simulink model "model5"  (R2022b)
settings: Solver=ode3  StartTime=0.0  StopTime=10  FixedStep=0.0005  RelTol=1e-3
values from neighbouring files (symbols this model uses):
  a21 = 1/2/m * x30^2 * FemP1/FemP2^2 * exp(-x10/FemP2)    [init.m]    (also in proj.m)
  a23 = -1/m * x30 * FemP1/FemP2 * exp(-x10/FemP2)    [init.m]    (also in proj.m)
  a31 = 1/f1 * exp(x10/f2) * (ki*u10 + ci - x30)    [init.m]    (also in proj.m)
  a33 = -f2/f1 * exp(x10/f2)    [init.m]    (also in proj.m)
  b31 = ki * f2/f1 * exp(x10/f2)    [init.m]    (also in proj.m)
  g = 9.81    [init.m]    (also in proj.m)
  K = place(A, B(:, 1), [-28, -60, -90])    [init.m]    (also in proj.m)
  L = acker(A', C', p)'    [init.m]    (also in proj.m)
  u10 = 1/ki*(x30-ci)    [init.m]    (also in proj.m)
  xd = d-bd    [init.m]    (also in proj.m)
settings Model: Creator=TheZl  LastModifiedBy=TheZl

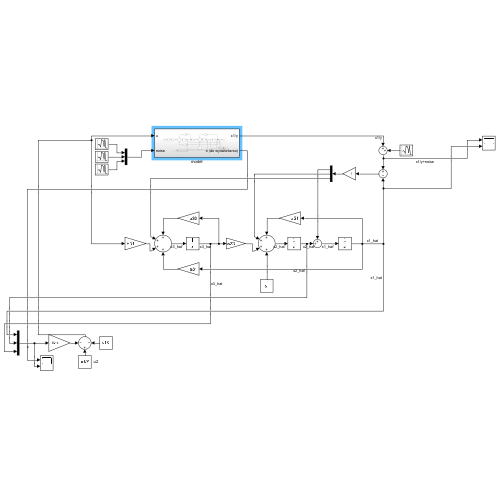
[thumbnail: Simulink's stored preview of the top-level diagram]
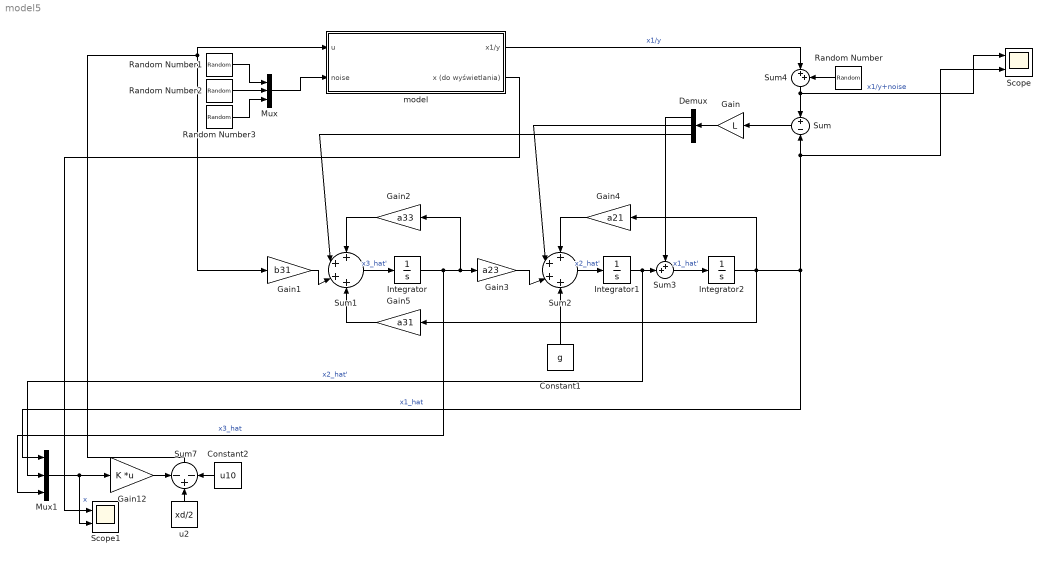
== system model5 ==
  Constant1 : Constant  Value=g
  Constant2 : Constant  Value=u10
  Demux : Demux  Outputs=3
  Gain : Gain  Gain=L
  Gain1 : Gain  Gain=b31
  Gain12 : Gain  Gain=K  Multiplication=Matrix(K*u)
  Gain2 : Gain  Gain=a33
  Gain3 : Gain  Gain=a23
  Gain4 : Gain  Gain=a21
  Gain5 : Gain  Gain=a31
  Integrator : Integrator
  Integrator1 : Integrator
  Integrator2 : Integrator  UpperSaturationLimit=xd  LowerSaturationLimit=0
  Mux : Mux  Inputs=3
  Mux1 : Mux  Inputs=3
  Random Number : RandomNumber  Variance=1e-5
  Random Number1 : RandomNumber  Variance=1e-5
  Random Number2 : RandomNumber  Variance=1e-5
  Random Number3 : RandomNumber  Variance=1e-2
  Scope : Scope  NumInputPorts=2
  Scope1 : Scope  NumInputPorts=2
  Sum : Sum  Inputs=+|-
  Sum1 : Sum  Inputs=++++
  Sum2 : Sum  Inputs=++++
  Sum3 : Sum  Inputs=++|
  Sum4 : Sum  Inputs=|++
  Sum7 : Sum  Inputs=-+-
  model : Subsystem
  u2 : Constant  Value=xd/2
  wires:
  model/1(x1/y) -> Sum4/1  "x1/y"
  Sum/1 -> Gain/1
  Sum7/1 -> Gain1/1, model/1(u)
  Gain4/1 -> Sum2/1
  Sum2/1 -> Integrator1/1  "x2_hat'"
  Sum1/1 -> Integrator/1  "x3_hat'"
  Constant1/1 -> Sum2/4
  Gain5/1 -> Sum1/4
  Gain2/1 -> Sum1/1
  Gain/1 -> Demux/1
  Demux/2 -> Sum2/2
  Gain3/1 -> Sum2/3
  Gain1/1 -> Sum1/3
  Sum3/1 -> Integrator2/1  "x1_hat'"
  Demux/1 -> Sum3/1
  Demux/3 -> Sum1/2
  Integrator2/1 -> Gain4/1, Mux1/1, Sum/2, Scope/2, Gain5/1  "x1_hat"
  Integrator/1 -> Mux1/3, Gain2/1, Gain3/1  "x3_hat"
  Integrator1/1 -> Mux1/2, Sum3/2  "x2_hat'"
  Gain12/1 -> Sum7/1
  Constant2/1 -> Sum7/3
  u2/1 -> Sum7/2
  Mux1/1 -> Scope1/2, Gain12/1  "x"
  Sum4/1 -> Sum/1, Scope/1  "x1/y+noise"
  Random Number/1 -> Sum4/2
  model/2(x (do wyświetlania)) -> Scope1/1
  Random Number1/1 -> Mux/1
  Mux/1 -> model/2(noise)
  Random Number2/1 -> Mux/2
  Random Number3/1 -> Mux/3

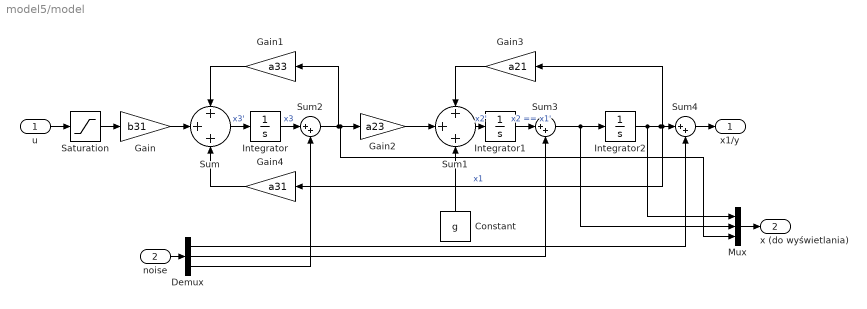
== system model5/model ==
  u : Inport
  noise : Inport  Port=2
  Constant : Constant  Value=g
  Demux : Demux  Outputs=3
  Gain : Gain  Gain=b31
  Gain1 : Gain  Gain=a33
  Gain2 : Gain  Gain=a23
  Gain3 : Gain  Gain=a21
  Gain4 : Gain  Gain=a31
  Integrator : Integrator
  Integrator1 : Integrator
  Integrator2 : Integrator  InitialCondition=xd  LimitOutput=on  UpperSaturationLimit=xd  LowerSaturationLimit=0
  Mux : Mux  Inputs=3
  Saturation : Saturate  UpperLimit=1  LowerLimit=0
  Sum : Sum  Inputs=+++
  Sum1 : Sum  Inputs=+++
  Sum2 : Sum  Inputs=|++
  Sum3 : Sum  Inputs=|++
  Sum4 : Sum  Inputs=|++
  x1/y : Outport
  x (do wyświetlania) : Outport  Port=2
  wires:
  Integrator2/1 -> Mux/1, Gain4/1, Gain3/1, Sum4/1  "x1"
  Gain1/1 -> Sum/1
  Integrator/1 -> Sum2/1  "x3"
  Constant/1 -> Sum1/3
  Gain/1 -> Sum/2
  Gain4/1 -> Sum/3
  u/1 -> Saturation/1
  Sum/1 -> Integrator/1  "x3'"
  Gain3/1 -> Sum1/1
  Sum1/1 -> Integrator1/1  "x2'"
  Saturation/1 -> Gain/1
  Gain2/1 -> Sum1/2
  Mux/1 -> x (do wyświetlania)/1
  Sum2/1 -> Mux/3, Gain2/1, Gain1/1
  Integrator1/1 -> Sum3/1  "x2 == x1'"
  Sum3/1 -> Mux/2, Integrator2/1
  Sum4/1 -> x1/y/1
  Demux/3 -> Sum2/2
  noise/1 -> Demux/1
  Demux/2 -> Sum3/2
  Demux/1 -> Sum4/2
